simulink model "SYS2_2"  (R2021b)
settings: Solver=VariableStepAuto  StartTime=0.0  StopTime=0.1  RelTol=1e-3
settings Model: Creator=Admin  LastModifiedBy=Admin

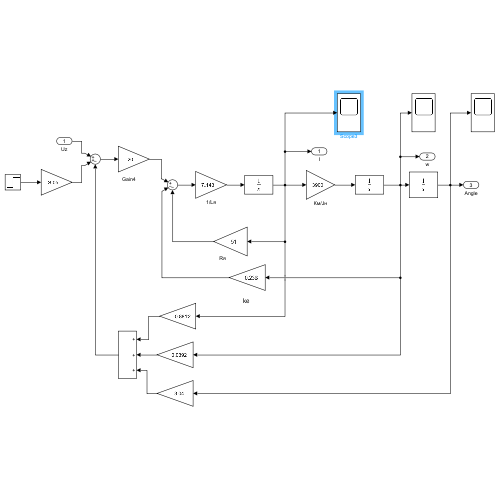
[thumbnail: Simulink's stored preview of the top-level diagram]
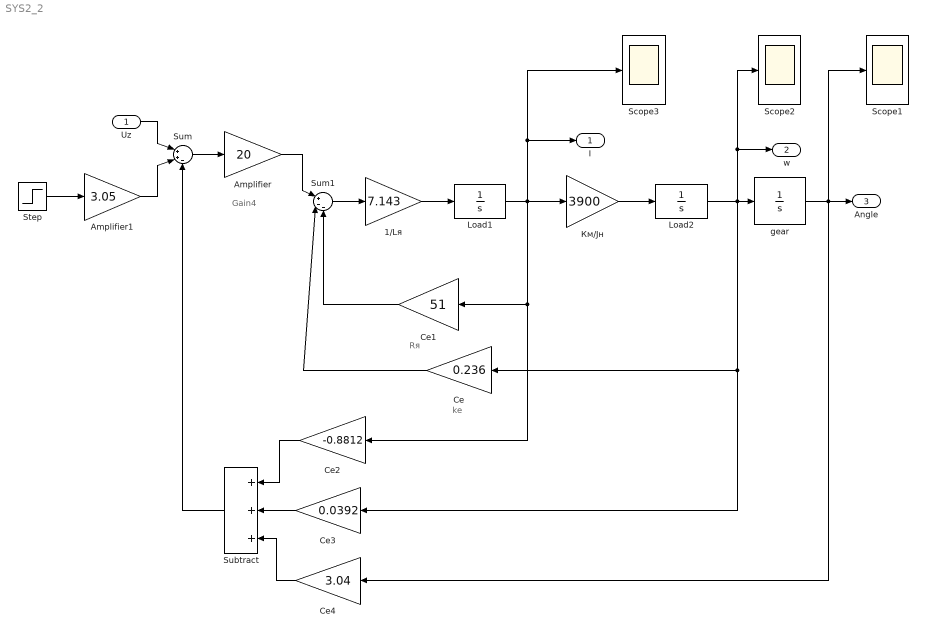
== system SYS2_2 ==
  note: Rя
  note: kе
  note: Gain4
  Uz : Inport
  1/Lя : Gain  Gain=7.143
  Amplifier : Gain  Gain=20
  Amplifier1 : Gain  Gain=3.05
  Ce : Gain  Gain=0.236
  Ce1 : Gain  Gain=51
  Ce2 : Gain  Gain=-0.8812
  Ce3 : Gain  Gain=0.0392
  Ce4 : Gain  Gain=3.04
  Load1 : TransferFcn  Denominator=[1 0]
  Load2 : TransferFcn  Denominator=[1 0]
  Scope1 : Scope
  Scope2 : Scope
  Scope3 : Scope
  Step : Step  Time=0  SampleTime=0
  Subtract : Sum  Inputs=+++
  Sum : Sum  Inputs=|++-
  Sum1 : Sum  Inputs=|+--
  gear : TransferFcn  Numerator=1  Denominator=[1 0]
  Км/Jн : Gain  Gain=3900
  I : Outport
  w : Outport  Port=2
  Angle : Outport  Port=3
  wires:
  Км/Jн/1 -> Load2/1
  Load2/1 -> Ce3/1, Ce/1, w/1, Scope2/1, gear/1
  Sum/1 -> Amplifier/1
  Sum1/1 -> 1/Lя/1
  Load1/1 -> I/1, Scope3/1, Км/Jн/1, Ce2/1, Ce1/1
  Uz/1 -> Sum/1
  Ce/1 -> Sum1/2
  Step/1 -> Amplifier1/1
  Ce1/1 -> Sum1/3
  1/Lя/1 -> Load1/1
  gear/1 -> Scope1/1, Ce4/1, Angle/1
  Amplifier/1 -> Sum1/1
  Amplifier1/1 -> Sum/2
  Ce2/1 -> Subtract/1
  Ce3/1 -> Subtract/2
  Ce4/1 -> Subtract/3
  Subtract/1 -> Sum/3
